simulink model "ARE_EDO"  (R2018b)
settings: Solver=VariableStepAuto  StartTime=0.0  StopTime=40  RelTol=1e-3
values from neighbouring files (symbols this model uses):
  Bz = [B ... (first row only)    [Dados.m]    (also in Dados_correct.m)
  Qz = [zeros(4,4), zeros(4,2) ... (first row only)    [Dados.m]    (also in Dados_correct.m; Function_ARE.m; areklmn_reactor.m; fd0.m)
  Rz = eye(2)    [Dados.m]    (also in Dados_correct.m)
settings Model: Creator=stayn  LastModifiedBy=Pendulo Rodas
settings DebuggingCC: LibraryContextMissingDiagnostic=none
settings SFSimCC: SimUseLocalCustomCode=off
settings RTWCC: RTWUseLocalCustomCode=off

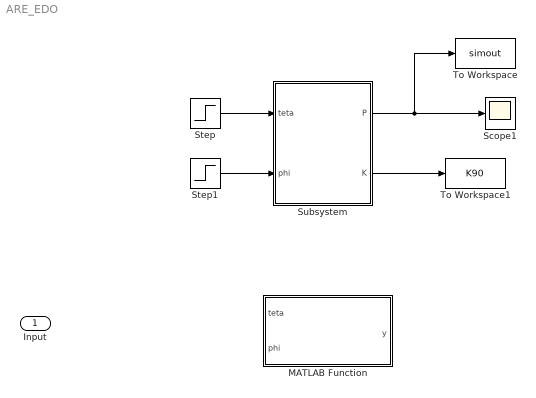
== system ARE_EDO ==
  Input : Inport
  MATLAB Function : MATLAB Function  TreatAsAtomicUnit=on
  Scope1 : Scope
  Step : Step  Time=5  After=1.570796  SampleTime=0
  Step1 : Step  Time=5  After=0  SampleTime=0
  Subsystem : Subsystem
  To Workspace : ToWorkspace  VariableName=simout  SaveFormat=Timeseries  SampleTime=0.1
  To Workspace1 : ToWorkspace  VariableName=K90  SaveFormat=Timeseries  SampleTime=-1
  wires:
  Subsystem/1(P) -> To Workspace/1, Scope1/1
  Step/1 -> Subsystem/1(teta)
  Step1/1 -> Subsystem/2("phi ")
  Subsystem/2(K) -> To Workspace1/1

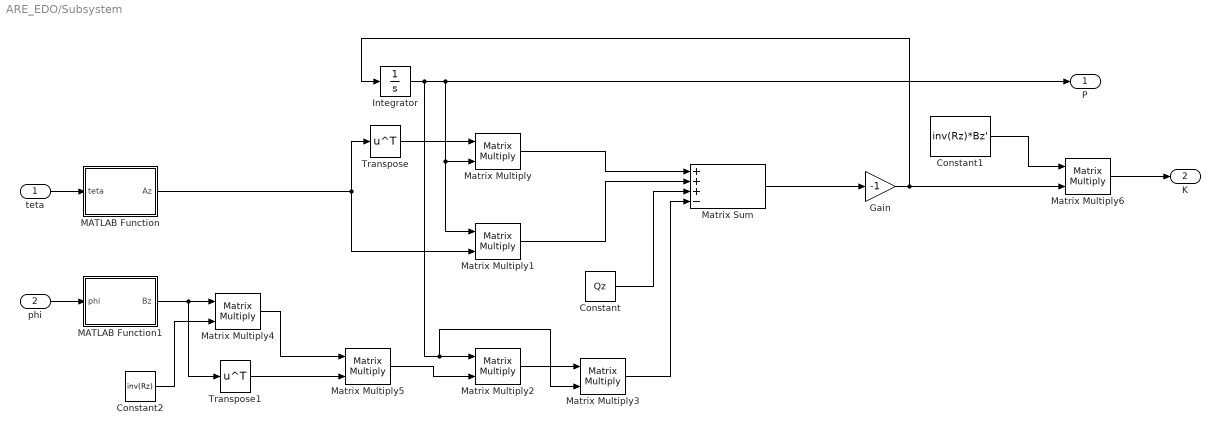
== system ARE_EDO/Subsystem ==
  teta : Inport
  "phi " : Inport  Port=2
  Constant : Constant  Value=Qz
  Constant1 : Constant  Value=inv(Rz)*Bz'
  Constant2 : Constant  Value=inv(Rz)
  Gain : Gain  Gain=-1
  Integrator : Integrator  IgnoreLimit=on
  MATLAB Function : MATLAB Function  TreatAsAtomicUnit=on
  MATLAB Function1 : MATLAB Function  TreatAsAtomicUnit=on
  Matrix Sum : Sum  Inputs=+++-
  Matrix Multiply{,1..6} (7 alike) : Product  Multiplication=Matrix(*)
  Transpose : Math  Operator=transpose  SaturateOnIntegerOverflow=on
  Transpose1 : Math  Operator=transpose  SaturateOnIntegerOverflow=on
  P : Outport
  K : Outport  Port=2
  wires:
  Gain/1 -> Matrix Multiply6/2, Integrator/1
  Integrator/1 -> Matrix Multiply3/2, Matrix Multiply2/1, Matrix Multiply/2, Matrix Multiply1/1, P/1
  Transpose1/1 -> Matrix Multiply5/2
  Matrix Multiply4/1 -> Matrix Multiply5/1
  teta/1 -> MATLAB Function/1(teta)
  Matrix Multiply6/1 -> K/1
  Constant/1 -> Matrix Sum/3
  Matrix Multiply5/1 -> Matrix Multiply2/2
  MATLAB Function1/1(Bz) -> Transpose1/1, Matrix Multiply4/1
  Matrix Multiply3/1 -> Matrix Sum/4
  Transpose/1 -> Matrix Multiply/1
  Matrix Multiply2/1 -> Matrix Multiply3/1
  Matrix Multiply1/1 -> Matrix Sum/2
  Matrix Sum/1 -> Gain/1
  MATLAB Function/1(Az) -> Transpose/1, Matrix Multiply1/2
  Constant1/1 -> Matrix Multiply6/1
  Constant2/1 -> Matrix Multiply4/2
  Matrix Multiply/1 -> Matrix Sum/1
  "phi "/1 -> MATLAB Function1/1(phi)

== matlab function ARE_EDO/Subsystem/MATLAB Function1 ==
  data: phi input; Bz output
function Bz = fcn(phi)

Jteta = 0.005425;    %1.0348 ;  (1/12*M*((b^2) + c^2)) + M*L1^2 
Jphi = 0.00201;  %0.0451;  (1/12*M*((2L^2) + c^2)) 
Kf = 0.056;      
% 0.0275;

L1 = 0.227          %0.227;
L2 = 0.08;

B = [ 0  0  ;
      Kf*L1/Jteta 0;
      0  0 ;
      0 Kf*L2/Jphi];
  
Bz = [B;
     zeros(2,2)];

== matlab function ARE_EDO/Subsystem/MATLAB Function ==
  data: teta input; Az output
function Az = fcn(teta)

Jteta = 0.005425;    %1.0348 ;  (1/12*M*((b^2) + c^2)) + M*L1^2 
Jphi = 0.00201;  %0.0451;  (1/12*M*((2L^2) + c^2)) 
Mh= 0.08;
Mw = 0.039;
Lw = 0.15;
g = 9.81;
L1 = 0.227 ;         %0.227;
c = 0.0076;
if teta == 0
    teta = 0.00001;
end
A = [  0  1  0  0;
      (Mw*g*Lw - Mh*g*L1)*sin(teta)/(teta*Jteta)   -c/Jteta  0  0;
       0  0  0  1;
       0  0  0  -c/Jphi];

D = [1 0 0 0;
     0 0 1 0];
  
 Az = [A, zeros(4,2)
      D, zeros(2,2)];

== matlab function ARE_EDO/MATLAB Function ==
  data: teta input; y output; phi input
function y=areklmn_reactor(teta,phi)
% STATE SPACE COEFFICIENT MATRICES
Jteta = 0.005425;    %(1/12*M*((b^2) + c^2)) + M*L1^2 
Jphi = 0.00201;   %(1/12*M*((2L^2) + c^2)) 
Kf = 0.056;      % 0.0275;
Mh= 0.08;
Mw = 0.039;
Lw = 0.15;
g = 9.81;
L1 = 0.227        
L2 = 0.08;
c = 0.0076;
L1 = 0.227;
L2 = 0.08;

A = [  0  1  0  0;
      (Mw*g*Lw - Mh*g*L1)*sin(teta)/Jteta   -c/Jteta  0  0;
       0  0  0  1;
       0  0  0  -c/Jphi];
B = [ 0  0  ;
      Kf*L1*cos(phi)/Jteta 0;
      0  0 ;
      0 Kf*L2/Jphi];
D = [1 0 0 0;
     0 0 1 0];
C = D;
% State weighting matrix and Control
Q=eye(4);
Q(1,1) = 20;
Q(3,3) = 10;
R=eye(2); % This value will be inverse of
A = [A, zeros(4,2)
          D, zeros(2,2)];
B = [B;
     zeros(2,2)];

Qz = [zeros(4,4), zeros(4,2)
      zeros(2,4), eye(2)];

Qz(5,5) = 20;   
Qz(6,6) = 1;

x10=rand([6,6]);

x0=[x10];
options = optimset('Display','iter','MaxFunEvals',50000000,'MaxIter' ,100,'TolFun',1e-6,'FunValCheck','on');
% fsolve to solve Algebric Riccati
figure(1)
x=fsolve(@areklmn_reactor,x0(:),options);

% Extracting elements from x to get
k=x(:);

% % Converting vectors into matrices
P=reshape(k,[6,6])

% Calculating Proportional term
K=inv(R)*B'*P
% Calculating Integral term
K1 = K(:,1:4);
K2 = K(:,5:6);

end

function y=areklmn_reactor(x,teta,phi)
Jteta = 0.005425;    %1.0348 ;  (1/12*M*((b^2) + c^2)) + M*L1^2 
Jphi = 0.00201;  %0.0451;  (1/12*M*((2L^2) + c^2)) 
Kf = 0.056;      
% 0.0275;
Mh= 0.08;
Mw = 0.039;
Lw = 0.15;
g = 9.81;
L1 = 0.227          %0.227;
L2 = 0.08;
c = 0.0076;
L1 = 0.227;
L2 = 0.08;

A = [  0  1  0  0;
      (Mw*g*Lw - Mh*g*L1)*sin(teta)/Jteta   -c/Jteta  0  0;
       0  0  0  1;
       0  0  0  -c/Jphi];
B = [ 0  0  ;
      Kf*L1*cos(phi)/Jteta 0;
      0  0 ;
      0 Kf*L2/Jphi];
  D = [1 0 0 0;
         0 0 1 0];
  
% State weighting matrix and Control
Q=eye(4);
Q(1,1) = 20;
Q(3,3) = 10;
R=eye(2); % This value will be inverse of
A = [A, zeros(4,2)
          D, zeros(2,2)];

    B = [B;
          zeros(2,2)];

    Qz = [zeros(4,4), zeros(4,2)
          zeros(2,4), eye(2)];

    Qz(5,5) = 20;   
    Qz(6,6) = 1;

% Extracting elements from x to get
P= reshape(x,[6,6])
% Converting vectors into matrices

% Four simultaneous nonlinear matrix
y= -A'*P - P*A - Qz + P*B*inv(R)*B'*P;
end
